simulink subsystem "Envelope"  (R2024a)
settings: Solver=VariableStepAuto  StartTime=0.0  StopTime=10.0  RelTol=1e-3
model mask{max_delay_sec=10}
  mask prompts: max_delay_sec "Maximum delay in seconds"
settings Model: Creator=david  LastModifiedBy=david

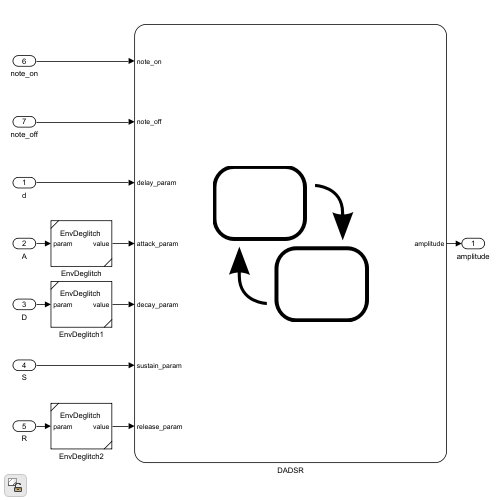
[thumbnail: Simulink's stored preview of the top-level diagram]
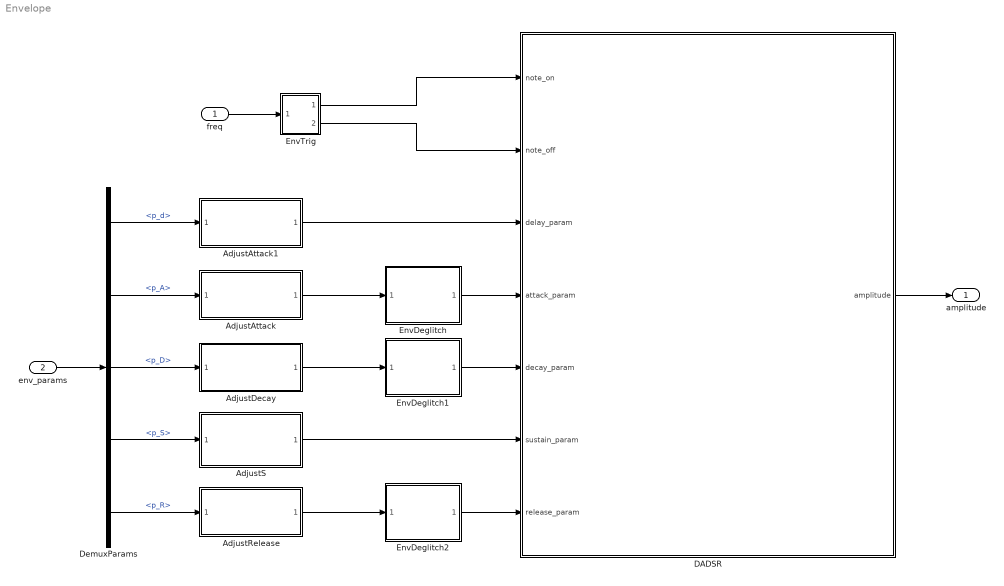
== system Envelope ==
  freq : Inport
  env_params : Inport  Port=2
  AdjustAttack : Subsystem  ReferencedSubsystem=AdjustEnvDelayParam
  AdjustAttack1 : Subsystem  ReferencedSubsystem=AdjustEnvDelayParam
  AdjustDecay : Subsystem  ReferencedSubsystem=AdjustEnvDelayParam
  AdjustRelease : Subsystem  ReferencedSubsystem=AdjustEnvDelayParam
  AdjustS : Subsystem  ReferencedSubsystem=AdjustEnvSustainParam
  DADSR : Stateflow chart  TreatAsAtomicUnit=on
  DemuxParams : BusSelector  OutputSignals=p_d,p_A,p_D,p_S,p_R
  EnvDeglitch : Subsystem  ReferencedSubsystem=EnvDeglitch
  EnvDeglitch1 : Subsystem  ReferencedSubsystem=EnvDeglitch
  EnvDeglitch2 : Subsystem  ReferencedSubsystem=EnvDeglitch
  EnvTrig : Subsystem
  amplitude : Outport
  wires:
  DemuxParams/2 -> AdjustAttack/1  "<p_A>"
  EnvDeglitch1/1 -> DADSR/5(decay_param)
  EnvDeglitch/1 -> DADSR/4(attack_param)
  EnvDeglitch2/1 -> DADSR/7(release_param)
  DemuxParams/3 -> AdjustDecay/1  "<p_D>"
  DemuxParams/4 -> AdjustS/1  "<p_S>"
  DemuxParams/5 -> AdjustRelease/1  "<p_R>"
  DADSR/1(amplitude) -> amplitude/1
  freq/1 -> EnvTrig/1(In1)
  EnvTrig/1(Out1) -> DADSR/1(note_on)
  EnvTrig/2(Out2) -> DADSR/2(note_off)
  env_params/1 -> DemuxParams/1
  AdjustAttack/1 -> EnvDeglitch/1
  AdjustDecay/1 -> EnvDeglitch1/1
  AdjustRelease/1 -> EnvDeglitch2/1
  AdjustS/1 -> DADSR/6(sustain_param)
  DemuxParams/1 -> AdjustAttack1/1  "<p_d>"
  AdjustAttack1/1 -> DADSR/3(delay_param)

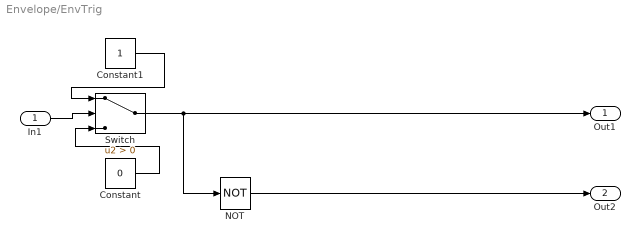
== system Envelope/EnvTrig ==
  In1 : Inport
  Constant : Constant  Value=0  OutDataTypeStr=boolean
  Constant1 : Constant  OutDataTypeStr=boolean
  NOT : Logic  Operator=NOT  IconShape=distinctive  AllPortsSameDT=off  OutDataTypeStr=boolean
  Switch : Switch  Criteria=u2 > Threshold  SaturateOnIntegerOverflow=off  InputSameDT=off
  Out1 : Outport
  Out2 : Outport  Port=2
  wires:
  Constant/1 -> Switch/3
  Constant1/1 -> Switch/1
  Switch/1 -> NOT/1, Out1/1
  In1/1 -> Switch/2
  NOT/1 -> Out2/1

== stateflow chart Envelope/DADSR ==
  state Pause
    entry:
    tk=0;
    amplitude=single(0);
  state Delay
    entry:
    tk=0;
    during:
    tk = tk+1;
  state Attack
    entry:
    amplitude = single(0);
    tk=0;
    during:
    amplitude = cincr(tk,attack_param,10,1);
    tk=tk + 1;
  state Decay
    entry:
    tk=0;
    max_amp=1-sustain_param;
    during:
    amplitude=1-cincr(tk,decay_param,10, max_amp);
    tk = tk+1;
  state Sustain
    entry:
    amplitude=sustain_param;
  state Release
    entry:
    tk=0;
    max_amp=amplitude;
    during:
    amplitude=max_amp-cincr(tk, release_param, 10, max_amp);
    tk=tk+1;
  (default) -> Pause
  Pause -> Delay : [note_on]
  Delay -> Pause [order 2] : [note_off]
  (junction 23) -> Pause
  Delay -> Attack [order 1] : [tk>=delay_param]
  Decay -> Sustain [order 1] : [tk>=decay_param]
  Attack -> Decay [order 1] : [tk==attack_param]
  Attack -> Release [order 2] : [note_off]
  Decay -> Release [order 2] : [note_off]
  Sustain -> Release : [note_off]
  Release -> (junction 23) : [tk==release_param]
  data: y function_output; t function_input; steps function_input; k function_input; max_amplitude function_input; note_on input; note_off input; tk local; delay_param input; attack_param input; decay_param input; amplitude output; sustain_param input; max_amp local; release_param input
  function y = cincr(t, steps, k, max_amplitude):
    | function y = cincr(t, steps, k, max_amplitude)
    |     y = single(max_amplitude * (1 - exp(-k * t/double(steps))));
    | end
